simulink model "method1"  (R2023b)
settings: Solver=ode4  StartTime=0.0  StopTime=10.0  FixedStep=0.001  RelTol=1e-3
InitFcn:
  | constants_pend
values from neighbouring files (symbols this model uses):
  f = 2    [constants_pend.m]    (also in formethod3.m = u(1))
  g = 9.81    [constants_pend.m]    (also in formethod3.m)
  initial = [0.5 , 5 , pi/3 , 0 ]    [constants_pend.m]
  l = 0.75    [constants_pend.m]    (also in formethod3.m)
  mc = 2    [constants_pend.m]    (also in formethod3.m)
  mp = 0.35    [constants_pend.m]    (also in formethod3.m)
settings Model: Creator=User  LastModifiedBy=User

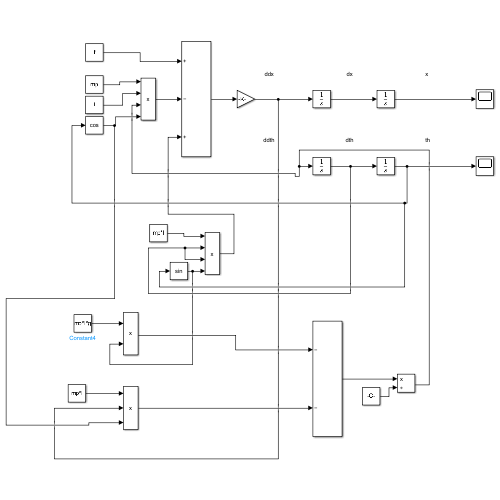
[thumbnail: Simulink's stored preview of the top-level diagram]
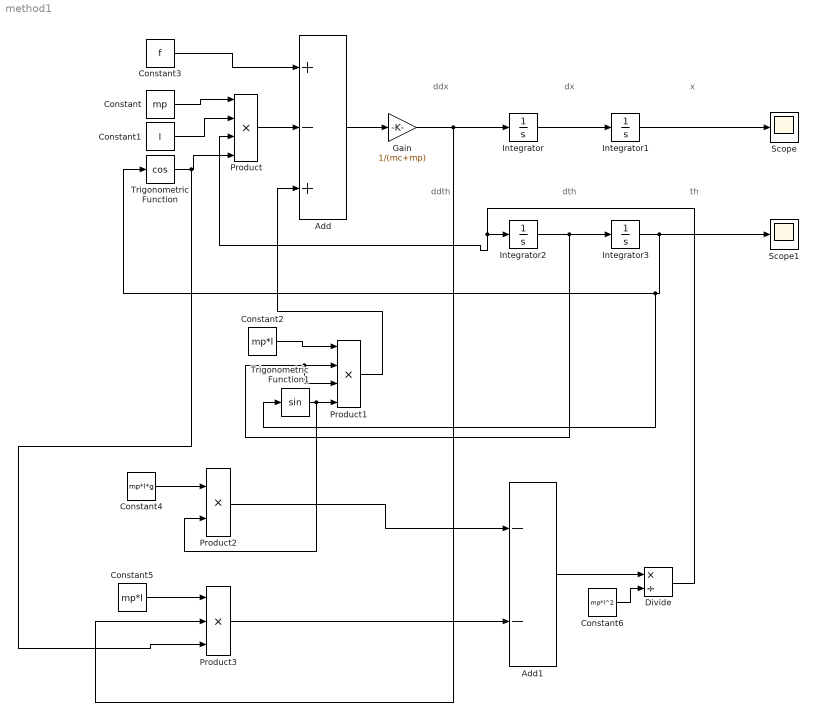
== system method1 ==
  note: th
  note: dth
  note: ddth
  note: x
  note: dx
  note: ddx
  Add : Sum  Inputs=+-+
  Add1 : Sum  Inputs=--
  Constant : Constant  Value=mp
  Constant1 : Constant  Value=l
  Constant2 : Constant  Value=mp*l
  Constant3 : Constant  Value=f
  Constant4 : Constant  Value=mp*l*g
  Constant5 : Constant  Value=mp*l
  Constant6 : Constant  Value=mp*l^2
  Divide : Product  Inputs=*/
  Gain : Gain  Gain=1/(mc+mp)
  Integrator : Integrator  InitialCondition=initial(2)
  Integrator1 : Integrator  InitialCondition=initial(1)
  Integrator2 : Integrator  InitialCondition=initial(4)
  Integrator3 : Integrator  InitialCondition=initial(3)
  Product : Product  Inputs=4
  Product1 : Product  Inputs=4
  Product2 : Product
  Product3 : Product  Inputs=3
  Scope : Scope
  Scope1 : Scope
  Trigonometric Function : Trigonometry  Operator=cos
  Trigonometric Function1 : Trigonometry
  wires:
  Integrator/1 -> Integrator1/1
  Integrator2/1 -> Product1/3, Product1/2, Integrator3/1
  Constant/1 -> Product/1
  Gain/1 -> Product3/2, Integrator/1
  Trigonometric Function/1 -> Product3/3, Product/4
  Constant1/1 -> Product/2
  Integrator3/1 -> Trigonometric Function1/1, Trigonometric Function/1, Scope1/1
  Constant2/1 -> Product1/1
  Trigonometric Function1/1 -> Product2/2, Product1/4
  Divide/1 -> Product/3, Integrator2/1
  Product/1 -> Add/2
  Constant3/1 -> Add/1
  Product1/1 -> Add/3
  Add/1 -> Gain/1
  Constant4/1 -> Product2/1
  Constant5/1 -> Product3/1
  Product2/1 -> Add1/1
  Product3/1 -> Add1/2
  Add1/1 -> Divide/1
  Constant6/1 -> Divide/2
  Integrator1/1 -> Scope/1
